simulink model "SeiralComm"  (R2022b)
settings: Solver=FixedStepAuto  StartTime=0.0  StopTime=10.0  FixedStep=1e-3  RelTol=1e-3  EnableMultiTasking=on
undefined symbols (not defined in the file): A0, A1, PTB2, PTB3
libraries: etargetslib x9, frdmk64flib x4
settings Model: ExtModeTrigDuration=5  Creator=hoang  LastModifiedBy=hoang
settings OptimizationCC: EnhancedBackFolding=on  PassReuseOutputArgsAs=Individual arguments  ZeroExternalMemoryAtStartup=off  ZeroInternalMemoryAtStartup=off  MaxStackSize=64  OptimizeBlockOrder=speed  DifferentSizesBufferReuse=on  OptimizationCustomize=off  EfficientTunableParamExpr=on
settings DebuggingCC: ParameterTunabilityLossMsg=error
settings HardwareCC: ProdBitPerPointer=32  ProdBitPerSizeT=32  ProdBitPerPtrDiffT=32  ProdLargestAtomicInteger=Long  ProdLargestAtomicFloat=Double  ProdWordSize=32  ProdHWDeviceType=ARM Compatible->ARM Cortex
settings ModelReferenceCC: EnableRefExpFcnMdlSchedulingChecks=on
settings SFSimCC: MATLABDynamicMemAlloc=off
settings RTWCC: Description=Embedded Coder  SystemTargetFile=ert.tlc  HardwareBoard=NXP FRDM-K64F  TLCOptions="-aInlineSetEventsForThisBaseRateFcn=TLC_FALSE -aSuppressMultiTaskScheduler=TLC_FALSE  -aRateBasedStepFcn=0"  TemplateMakefile=ert_default_tmf  Toolchain=GNU Tools for ARM Embedded Processors
settings CodeAppCC: ForceParamTrailComments=on  IgnoreCustomStorageClasses=off  OperatorAnnotations=on  SimulinkDataObjDesc=on  SFDataObjDesc=on  InsertBlockDesc=on
settings ERTTargetCC: ExtModeTransport=4  ExtModeMexFile=sendToCommService

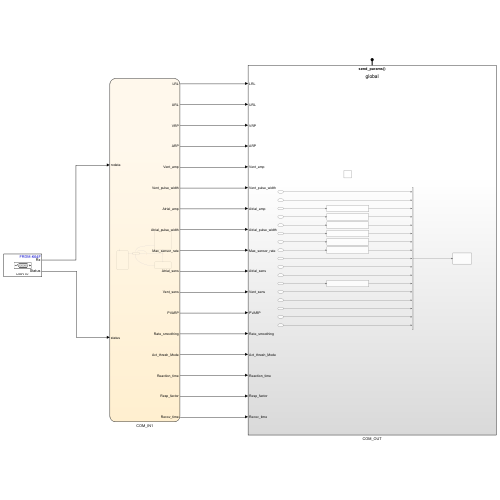
[thumbnail: Simulink's stored preview of the top-level diagram]
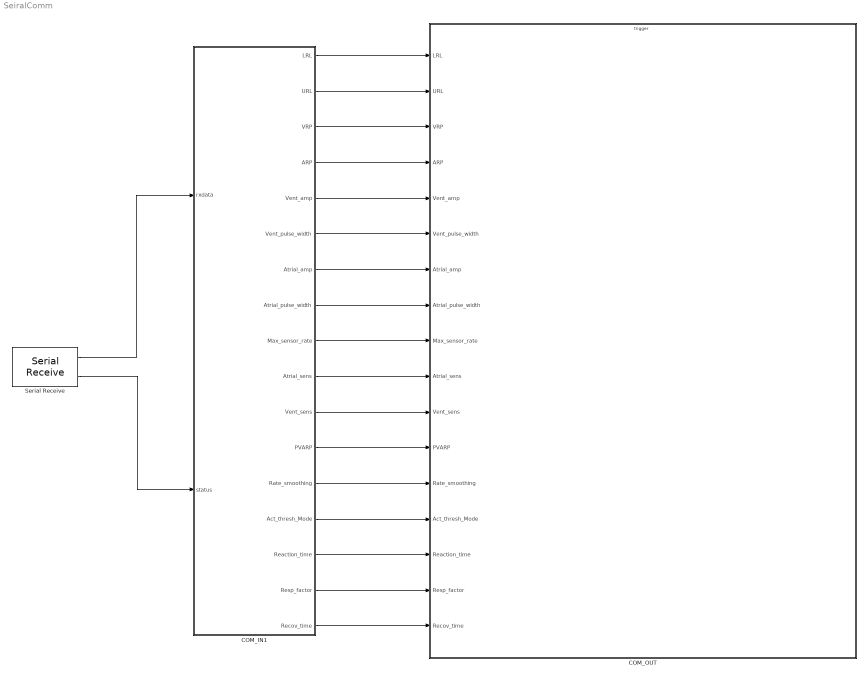
== system SeiralComm ==
  COM_IN1 : Stateflow chart  TreatAsAtomicUnit=on
  COM_OUT : Subsystem
  Serial Receive : frdmk64flib/Serial Receive  SCIModule=0  Baudrate=uint32(9600)  Parity=None  StopBits=1  HardwareFlowControl=None  ByteOrder=LittleEndian  DataType=uint8  DataLength=10  BlockingMode=off  OutputStatus=on  SampleTime=0.1
  wires:
  Serial Receive/1 -> COM_IN1/1(rxdata)
  Serial Receive/2 -> COM_IN1/2(status)
  COM_IN1/1(LRL) -> COM_OUT/1(LRL)
  COM_IN1/2(URL) -> COM_OUT/2(URL)
  COM_IN1/3(VRP) -> COM_OUT/3(VRP)
  COM_IN1/4(ARP) -> COM_OUT/4(ARP)
  COM_IN1/5(Vent_amp) -> COM_OUT/5(Vent_amp)
  COM_IN1/6(Vent_pulse_width) -> COM_OUT/6(Vent_pulse_width)
  COM_IN1/7(Atrial_amp) -> COM_OUT/7(Atrial_amp)
  COM_IN1/8(Atrial_pulse_width) -> COM_OUT/8(Atrial_pulse_width)
  COM_IN1/9(Max_sensor_rate) -> COM_OUT/9(Max_sensor_rate)
  COM_IN1/10(Atrial_sens) -> COM_OUT/10(Atrial_sens)
  COM_IN1/11(Vent_sens) -> COM_OUT/11(Vent_sens)
  COM_IN1/12(PVARP) -> COM_OUT/12(PVARP)
  COM_IN1/13(Rate_smoothing) -> COM_OUT/13(Rate_smoothing)
  COM_IN1/14(Act_thresh_Mode) -> COM_OUT/14(Act_thresh_Mode)
  COM_IN1/15(Reaction_time) -> COM_OUT/15(Reaction_time)
  COM_IN1/16(Resp_factor) -> COM_OUT/16(Resp_factor)
  COM_IN1/17(Recov_time) -> COM_OUT/17(Recov_time)

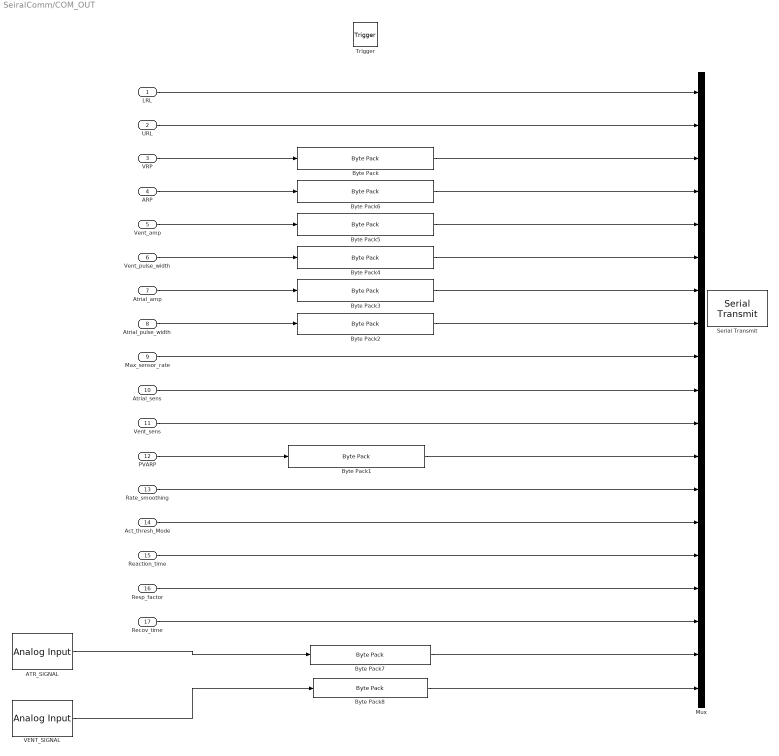
== system SeiralComm/COM_OUT ==
  LRL : Inport  OutDataTypeStr=uint8
  URL : Inport  Port=2  OutDataTypeStr=uint8
  VRP : Inport  Port=3  OutDataTypeStr=single
  ARP : Inport  Port=4  OutDataTypeStr=single
  Vent_amp : Inport  Port=5  OutDataTypeStr=single
  Vent_pulse_width : Inport  Port=6  OutDataTypeStr=single
  Atrial_amp : Inport  Port=7  OutDataTypeStr=int16
  Atrial_pulse_width : Inport  Port=8  OutDataTypeStr=int16
  Max_sensor_rate : Inport  Port=9  OutDataTypeStr=uint8
  Atrial_sens : Inport  Port=10  OutDataTypeStr=uint8
  Vent_sens : Inport  Port=11  OutDataTypeStr=uint8
  PVARP : Inport  Port=12  OutDataTypeStr=int16
  Rate_smoothing : Inport  Port=13  OutDataTypeStr=uint8
  Act_thresh_Mode : Inport  Port=14  OutDataTypeStr=uint8
  Reaction_time : Inport  Port=15  OutDataTypeStr=uint8
  Resp_factor : Inport  Port=16  OutDataTypeStr=uint8
  Recov_time : Inport  Port=17  OutDataTypeStr=uint8
  Trigger : TriggerPort  TriggerType=function-call  IsSimulinkFunction=on  FunctionName=send_params  VariantControl=(inherit)  PortDimensions=1
  ATR_SIGNAL : frdmk64flib/Analog Input  Whichpin=PTB2 (A0)  SampleTime=-1
  Byte Pack{,4..6} (4 alike) : etargetslib/Byte Pack  datatypes={'single'}  byteAlign=1
  Byte Pack1 : etargetslib/Byte Pack  datatypes={'int16'}  byteAlign=1
  Byte Pack2 : etargetslib/Byte Pack  datatypes={'int16'}  byteAlign=1
  Byte Pack3 : etargetslib/Byte Pack  datatypes={'int16'}  byteAlign=1
  Byte Pack7 : etargetslib/Byte Pack  datatypes={'double'}  byteAlign=1
  Byte Pack8 : etargetslib/Byte Pack  datatypes={'double'}  byteAlign=1
  Mux : Mux  Inputs=19
  Serial Transmit : frdmk64flib/Serial Transmit  SCIModule=0  Baudrate=uint32(9600)  Parity=None  StopBits=1  HardwareFlowControl=None  ByteOrder=LittleEndian  BlockingMode=on  OutputStatus=off
  VENT_SIGNAL : frdmk64flib/Analog Input  Whichpin=PTB3 (A1)  SampleTime=-1
  wires:
  PVARP/1 -> Byte Pack1/1
  VRP/1 -> Byte Pack/1
  ARP/1 -> Byte Pack6/1
  Vent_amp/1 -> Byte Pack5/1
  Vent_pulse_width/1 -> Byte Pack4/1
  Atrial_amp/1 -> Byte Pack3/1
  Atrial_pulse_width/1 -> Byte Pack2/1
  ATR_SIGNAL/1 -> Byte Pack7/1
  VENT_SIGNAL/1 -> Byte Pack8/1
  LRL/1 -> Mux/1
  URL/1 -> Mux/2
  Byte Pack/1 -> Mux/3
  Byte Pack6/1 -> Mux/4
  Byte Pack5/1 -> Mux/5
  Byte Pack4/1 -> Mux/6
  Byte Pack3/1 -> Mux/7
  Byte Pack2/1 -> Mux/8
  Max_sensor_rate/1 -> Mux/9
  Atrial_sens/1 -> Mux/10
  Vent_sens/1 -> Mux/11
  Byte Pack1/1 -> Mux/12
  Recov_time/1 -> Mux/17
  Resp_factor/1 -> Mux/16
  Reaction_time/1 -> Mux/15
  Act_thresh_Mode/1 -> Mux/14
  Rate_smoothing/1 -> Mux/13
  Byte Pack7/1 -> Mux/18
  Byte Pack8/1 -> Mux/19

== stateflow chart SeiralComm/COM_IN1 ==
  state SET_PARAM
    entry:
    LRL = rxdata(3);
    URL = rxdata(4);
    Atrial_amp = typecast(rxdata(5:8), 'single');
    Atrial_pulse_width = typecast(rxdata(9:12), 'single');
    Vent_amp = typecast(rxdata(13:16), 'single');
    Vent_pulse_width = typecast(rxdata(17:20), 'single');
    VRP = typecast(rxdata(21:22), 'int16');
    ARP = typecast(rxdata(23:24), 'int16');
    Max_sensor_rate = cast(rxdata(25), 'uint8');
    Atrial_sens = cast(rxdata(26), 'uint8');
    Vent_sens = cast(rxdata(27), 'uint8');
    PVARP = typecast(rxdata(28:29), 'int16');
    Rate_smoothing = cast(rxdata(30), 'uint8');
    Act_thresh_Mode = cast(rxdata(31), 'uint8');
    Reaction_time = cast(rxdata(32), 'uint8');
    Resp_factor = cast(rxdata(33), 'uint8');
    Recov_time = cast(rxdata(34), 'uint8');
  state INITIAL
    entry:
    LRL = 30; %ppm
    URL = 50; %ppm
    Atrial_amp = 0;
    Atrial_pulse_width = 0.05;
    Vent_amp = 0;
    Vent_pulse_width = 0.05;
    VRP = 150;
    ARP = 150;
    Max_sensor_rate = 50;
    Atrial_sens = 0;
    Vent_sens = 0;
    PVARP = 10;
    Rate_smoothing = 0;
    Act_thresh_Mode = 0;
    Reaction_time = 10;
    Resp_factor = 1;
    Recov_time = 2;
  state STANDBY
    %waiting for COM
  state ECHO_PARAM
    entry:
    send_params();
  SET_PARAM -> STANDBY
  (default) -> INITIAL
  (junction 14) -> SET_PARAM [order 1] : [rxdata(2) == hex2dec('55')]
  INITIAL -> STANDBY
  STANDBY -> (junction 15) : [status == 0]
  (junction 15) -> (junction 14) : [rxdata(1) == hex2dec('16')]
  (junction 14) -> ECHO_PARAM [order 2] : [rxdata(2) == hex2dec('22')]
  ECHO_PARAM -> STANDBY
  data: rxdata input uint8; status input uint8; LRL output uint8; URL output uint8; VRP output single; ARP output single; Vent_amp output single; Vent_pulse_width output single; Atrial_amp output int16; Atrial_pulse_width output int16; Max_sensor_rate output uint8; Atrial_sens output uint8; Vent_sens output uint8; PVARP output int16; Rate_smoothing output uint8; Act_thresh_Mode output uint8; Reaction_time output uint8; Resp_factor output uint8; Recov_time output uint8
